simulink model "DPF_WARNING_LAMP"  (R2018a)
settings: Solver=VariableStepAuto  StartTime=0.0  StopTime=110  RelTol=1e-3
undefined symbols (not defined in the file or in its folder): Delta_presure, T2
libraries: simulink x6, powerlib_meascontrol x1
settings Model: Creator=Home  LastModifiedBy=Home

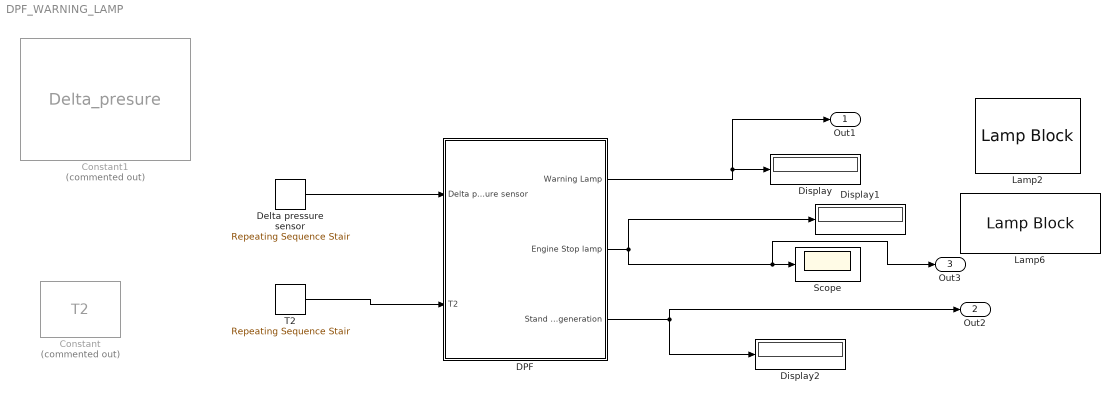
== system DPF_WARNING_LAMP ==
  Constant : Constant  Commented=on  Value=T2
  Constant1 : Constant  Commented=on  Value=Delta_presure
  DPF : Subsystem
  Delta pressure sensor : simulink/Sources/Repeating Sequence Stair  OutValues=[0 0.1 0.2 0.4 0.8 0.9 1].'  tsamp=-1  OutMin=[]  OutMax=[]  OutDataTypeStr=double  OutputDataTypeScalingMode=double  OutDataType=fixdt(0,8)  ConRadixGroup=Best Precision: Vector-wise  OutScaling=2^-12
  Display : Display
  Display1 : Display
  Display2 : Display
  Lamp2 : LampBlock  WebBlockId=17
  Lamp6 : LampBlock  WebBlockId=22
  Scope : Scope
  T2 : simulink/Sources/Repeating Sequence Stair  OutValues=[200 300 400 500 600].'  tsamp=-1  OutMin=[]  OutMax=[]  OutDataTypeStr=double  OutputDataTypeScalingMode=double  OutDataType=fixdt(0,8)  ConRadixGroup=Best Precision: Vector-wise  OutScaling=2^-12
  Out1 : Outport
  Out2 : Outport  Port=2
  Out3 : Outport  Port=3
  wires:
  DPF/1(Warning Lamp) -> Out1/1, Display/1
  DPF/2(Engine Stop lamp) -> Display1/1, Out3/1, Scope/1
  DPF/3("Stand still regeneration ") -> Out2/1, Display2/1
  Delta pressure sensor/1 -> DPF/1(Delta pressure sensor)
  T2/1 -> DPF/2("T2 ")

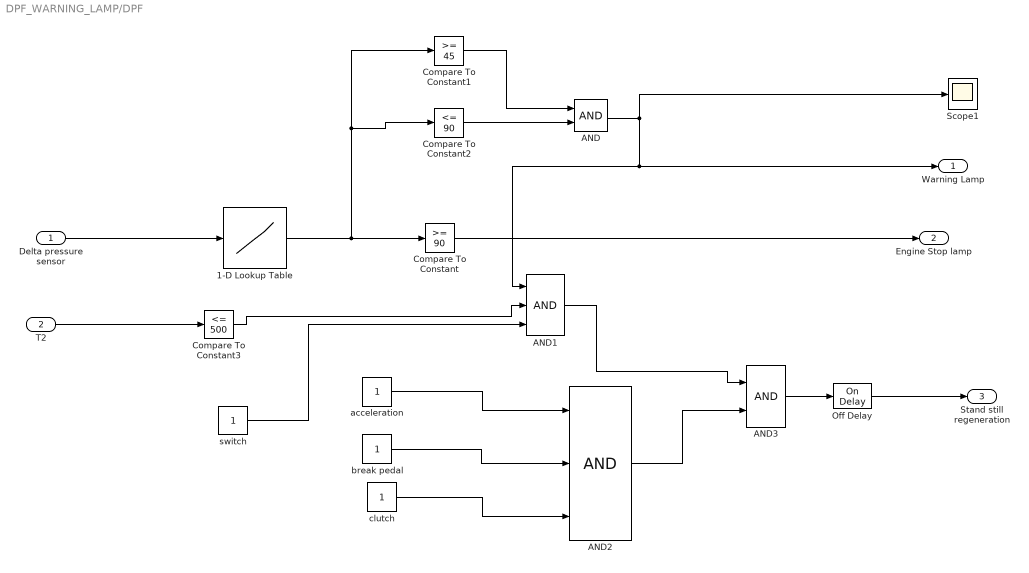
== system DPF_WARNING_LAMP/DPF ==
  Delta pressure sensor : Inport
  "T2 " : Inport  Port=2
  1-D Lookup Table : Lookup_n-D  NumberOfTableDimensions=1  BreakpointsForDimension1=[0:0.1:1]  Table=[0:10:100]  InternalRulePriority=Speed  RndMeth=Simplest  InputSameDT=on
  AND : Logic  AllPortsSameDT=off  OutDataTypeStr=boolean
  AND1 : Logic  Inputs=3  AllPortsSameDT=off  OutDataTypeStr=boolean
  AND2 : Logic  Inputs=3  AllPortsSameDT=off  OutDataTypeStr=boolean
  AND3 : Logic  AllPortsSameDT=off  OutDataTypeStr=boolean
  Compare To Constant : simulink/Logic and Bit Operations/Compare To Constant  relop=>=  const=90  OutDataTypeStr=boolean
  Compare To Constant1 : simulink/Logic and Bit Operations/Compare To Constant  relop=>=  const=45  OutDataTypeStr=boolean
  Compare To Constant2 : simulink/Logic and Bit Operations/Compare To Constant  relop=<=  const=90  OutDataTypeStr=boolean
  Compare To Constant3 : simulink/Logic and Bit Operations/Compare To Constant  relop=<=  const=500  OutDataTypeStr=boolean
  Off Delay : powerlib_meascontrol/Logic/On Delay  DelayType=Off delay  delay=1800  ic=1  Ts=0
      settings: SourceProductName=Simscape Power Systems
  Scope1 : Scope
  acceleration : Constant
  break pedal : Constant
  clutch : Constant
  switch : Constant
  Warning Lamp : Outport
  Engine Stop lamp : Outport  Port=2
  "Stand still regeneration " : Outport  Port=3
  wires:
  break pedal/1 -> AND2/2
  clutch/1 -> AND2/3
  AND/1 -> Scope1/1, Warning Lamp/1, AND1/1
  1-D Lookup Table/1 -> Compare To Constant2/1, Compare To Constant1/1, Compare To Constant/1
  Compare To Constant1/1 -> AND/1
  Compare To Constant3/1 -> AND1/2
  switch/1 -> AND1/3
  AND2/1 -> AND3/2
  Off Delay/1 -> "Stand still regeneration "/1
  Compare To Constant2/1 -> AND/2
  AND1/1 -> AND3/1
  AND3/1 -> Off Delay/1
  acceleration/1 -> AND2/1
  "T2 "/1 -> Compare To Constant3/1
  Delta pressure sensor/1 -> 1-D Lookup Table/1
  Compare To Constant/1 -> Engine Stop lamp/1
